simulink model "model_R2019b"  (R2021b)
settings: Solver=FixedStepDiscrete  StartTime=0.0  StopTime=inf  FixedStep=5e-3  RelTol=1e-3
values from neighbouring files (symbols this model uses):
  emin = 0.5    [simulate.m]
  gamma = 0.3    [simulate.m]
  k = 1    [simulate.m]
  omega_max = (pi/180)*300    (= 5.23598775598)    [simulate.m]
  u_max = 1.2    [simulate.m]
libraries: fuzblock x2, simulink x1
settings Model: Creator=mateu  LastModifiedBy=breno-meneses
settings SolverCC: AlgebraicLoopSolver=TrustRegion
settings DebuggingCC: UnconnectedInputMsg=none  UnconnectedOutputMsg=none  UnconnectedLineMsg=none

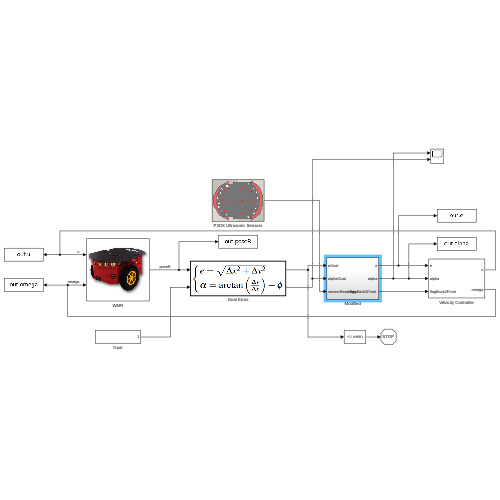
[thumbnail: Simulink's stored preview of the top-level diagram]
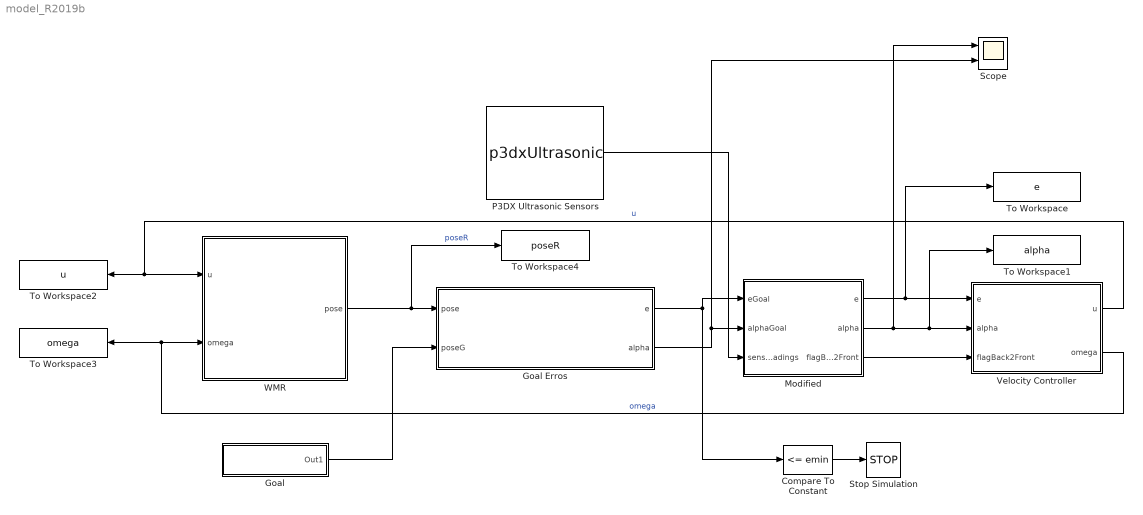
== system model_R2019b ==
  Compare To Constant : simulink/Logic and Bit Operations/Compare To Constant  relop=<=  const=emin  OutDataTypeStr=boolean
  Goal : Subsystem  VariantControl=GOAL_COPPELIA
  Goal Erros : MATLAB Function  TreatAsAtomicUnit=on
  Modified : Subsystem  VariantControl=BC_MODIFIED
  P3DX Ultrasonic Sensors : M-S-Function  FunctionName=p3dxUltrasonic
      mask Display: image('$imagefile'); % Use "Edit Image" on toolstrip to change.
  Scope : Scope  NumInputPorts=2
  Stop Simulation : Stop
  To Workspace : ToWorkspace  VariableName=e  SaveFormat=Timeseries  SampleTime=-1
  To Workspace1 : ToWorkspace  VariableName=alpha  SaveFormat=Timeseries  SampleTime=-1
  To Workspace2 : ToWorkspace  VariableName=u  SaveFormat=Timeseries  SampleTime=-1
  To Workspace3 : ToWorkspace  VariableName=omega  SaveFormat=Timeseries  SampleTime=-1
  To Workspace4 : ToWorkspace  VariableName=poseR  SaveFormat=Timeseries  SampleTime=-1
  Velocity Controller : Subsystem
  WMR : Subsystem  VariantControl=UNICYCLE_COPPELIA
      mask Display: image('$imagefile'); % Use "Edit Image" on toolstrip to change.
  wires:
  WMR/1(pose) -> To Workspace4/1, Goal Erros/1(pose)  "poseR"
  Goal/1(Out1) -> Goal Erros/2(poseG)
  Compare To Constant/1 -> Stop Simulation/1
  Velocity Controller/1(u) -> WMR/1(u), To Workspace2/1  "u"
  Velocity Controller/2(omega) -> WMR/2(omega), To Workspace3/1  "omega"
  Modified/1(e) -> Velocity Controller/1(e), To Workspace/1
  Modified/2(alpha) -> Velocity Controller/2(alpha), To Workspace1/1, Scope/1
  Goal Erros/1(e) -> Modified/1(eGoal), Compare To Constant/1
  Goal Erros/2(alpha) -> Scope/2, Modified/2(alphaGoal)
  P3DX Ultrasonic Sensors/1 -> Modified/3(sensorReadings)
  Modified/3("flagBack2Front ") -> Velocity Controller/3("flagBack2Front ")

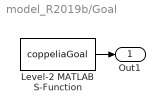
== system model_R2019b/Goal ==
  Level-2 MATLAB S-Function : M-S-Function  FunctionName=coppeliaGoal
  Out1 : Outport
  wires:
  Level-2 MATLAB S-Function/1 -> Out1/1

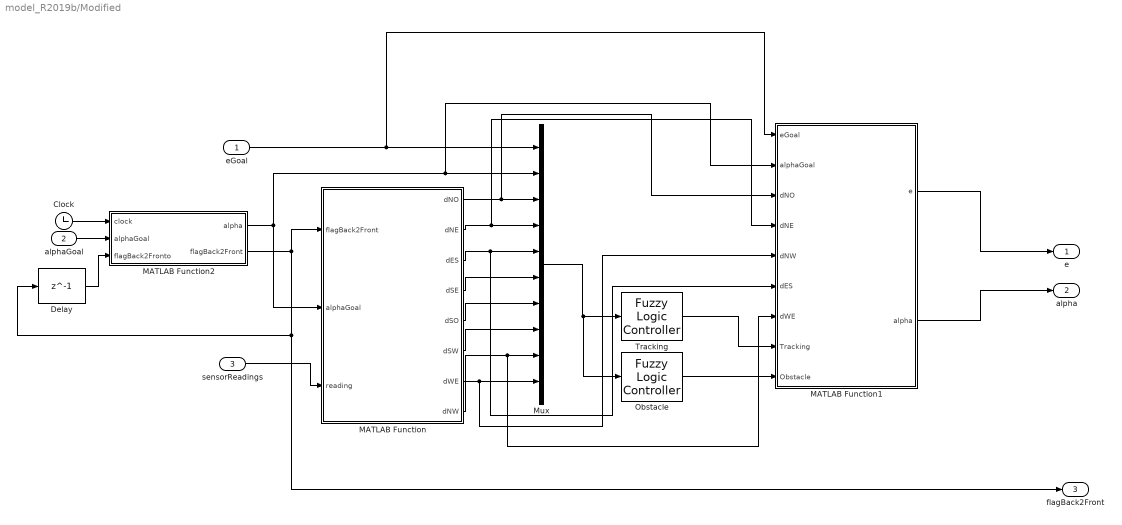
== system model_R2019b/Modified ==
  eGoal : Inport
  alphaGoal : Inport  Port=2
  sensorReadings : Inport  Port=3
  Clock : Clock
  Delay : Delay  DelayLength=1  InputProcessing=Columns as channels (frame based)
  MATLAB Function : MATLAB Function  TreatAsAtomicUnit=on
  MATLAB Function1 : MATLAB Function  TreatAsAtomicUnit=on
  MATLAB Function2 : MATLAB Function  TreatAsAtomicUnit=on
  Mux : Mux  Inputs=10
  "Obstacle " : fuzblock/Fuzzy Logic  Controller  FIS=Obstacle  OutputSampleNumber=101  DataType=double  FuzzifiedInputs=off  RuleFiringStrengths=off  RuleOutputs=off  AggregatedOutputs=off  SimulateUsing=Interpreted execution  OutOfRangeInputValueMessage=warning  NoRuleFiredMessage=warning  EmptyOutputFuzzySetMessage=warning
  Tracking : fuzblock/Fuzzy Logic  Controller  FIS=Tracking  OutputSampleNumber=101  DataType=double  FuzzifiedInputs=off  RuleFiringStrengths=off  RuleOutputs=off  AggregatedOutputs=off  SimulateUsing=Interpreted execution  OutOfRangeInputValueMessage=warning  NoRuleFiredMessage=warning  EmptyOutputFuzzySetMessage=warning
  e : Outport
  alpha : Outport  Port=2
  "flagBack2Front " : Outport  Port=3
  wires:
  sensorReadings/1 -> MATLAB Function/3(reading)
  MATLAB Function/1(dNO) -> MATLAB Function1/3(dNO), Mux/3
  MATLAB Function/2(dNE) -> MATLAB Function1/4(dNE), Mux/4
  MATLAB Function/3(dES) -> MATLAB Function1/6(dES), Mux/5
  MATLAB Function/4(dSE) -> Mux/6
  MATLAB Function/5(dSO) -> Mux/7
  MATLAB Function/6(dSW) -> Mux/8
  MATLAB Function/7(dWE) -> MATLAB Function1/7(dWE), Mux/9
  MATLAB Function/8(dNW) -> MATLAB Function1/5(dNW), Mux/10
  eGoal/1 -> MATLAB Function1/1(eGoal), Mux/1
  MATLAB Function1/2(alpha) -> alpha/1
  MATLAB Function1/1(e) -> e/1
  Tracking/1 -> MATLAB Function1/8(Tracking)
  MATLAB Function2/1(alpha) -> MATLAB Function/2(alphaGoal), MATLAB Function1/2(alphaGoal), Mux/2
  "Obstacle "/1 -> MATLAB Function1/9(Obstacle)
  Mux/1 -> "Obstacle "/1, Tracking/1
  MATLAB Function2/2(flagBack2Front) -> Delay/1, "flagBack2Front "/1, MATLAB Function/1(flagBack2Front)
  alphaGoal/1 -> MATLAB Function2/2(alphaGoal)
  Clock/1 -> MATLAB Function2/1(clock)
  Delay/1 -> MATLAB Function2/3(flagBack2Fronto)

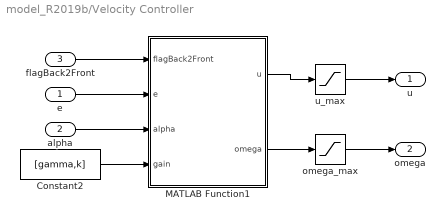
== system model_R2019b/Velocity Controller ==
  e : Inport
  alpha : Inport  Port=2
  "flagBack2Front " : Inport  Port=3
  Constant2 : Constant  Value=[gamma,k]
  MATLAB Function1 : MATLAB Function  TreatAsAtomicUnit=on
  omega_max : Saturate  UpperLimit=omega_max  LowerLimit=-omega_max
  u_max : Saturate  UpperLimit=u_max  LowerLimit=-u_max
  u : Outport
  omega : Outport  Port=2
  wires:
  Constant2/1 -> MATLAB Function1/4(gain)
  omega_max/1 -> omega/1
  u_max/1 -> u/1
  alpha/1 -> MATLAB Function1/3(alpha)
  e/1 -> MATLAB Function1/2(e)
  MATLAB Function1/2(omega) -> omega_max/1
  MATLAB Function1/1(u) -> u_max/1
  "flagBack2Front "/1 -> MATLAB Function1/1(flagBack2Front)

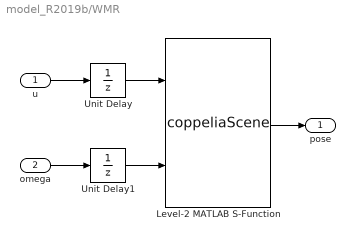
== system model_R2019b/WMR ==
  u : Inport
  omega : Inport  Port=2
  Level-2 MATLAB S-Function : M-S-Function  FunctionName=coppeliaScene
  Unit Delay : UnitDelay  SampleTime=-1  HasFrameUpgradeWarning=on
  Unit Delay1 : UnitDelay  SampleTime=-1  HasFrameUpgradeWarning=on
  pose : Outport
  wires:
  u/1 -> Unit Delay/1
  omega/1 -> Unit Delay1/1
  Level-2 MATLAB S-Function/1 -> pose/1
  Unit Delay/1 -> Level-2 MATLAB S-Function/1
  Unit Delay1/1 -> Level-2 MATLAB S-Function/2

== matlab function model_R2019b/Modified/MATLAB Function ==
  data: flagBack2Front input; alphaGoal input; reading input; dNO output; dNE output; dES output; dSE output; dSO output; dSW output; dWE output; dNW output
function [dNO,dNE,dES,dSE,dSO,dSW,dWE,dNW] = getDistances(flagBack2Front,alphaGoal,reading)

    
if(flagBack2Front)
    dNO = min(reading(12:13));
    dSO = min(reading(4:5));
    dES = min([reading(1),reading(16)]);
    dWE = min(reading(8:9));
    dSE = min(reading(2:3));
    dNW = min(reading(10:11));
    dNE = min(reading(14:15)); 
    dSW = min(reading(6:7));
else
    dNO = min(reading(4:5));
    dSO = min(reading(12:13));
    dES = min(reading(8:9));
    dWE = min([reading(1),reading(16)]);
    dSE = min(reading(10:11));
    dNW = min(reading(2:3));
    dNE = min(reading(6:7));
    dSW = min(reading(14:15));
end

end

== matlab function model_R2019b/Goal Erros ==
  settings: updateMethod=DISCRETE  sampleTime=0.05
  data: pose input; e output; poseG input; alpha output
function [e,alpha] = errors(pose,poseG)

deltaX = poseG(1)-pose(1); deltaY = poseG(2)-pose(2);
phi = pose(3);

e = sqrt(deltaX^2 + deltaY^2);
alpha = atan2(deltaY,deltaX) - phi;

if alpha < -pi
    alpha = alpha + 2*pi;
elseif alpha >= pi
    alpha = alpha - 2*pi;
end

== matlab function model_R2019b/Velocity Controller/MATLAB Function1 ==
  settings: updateMethod=DISCRETE  sampleTime=0.05
  data: flagBack2Front input; e input; u output; alpha input; omega output; gain input
function [u,omega] = control(flagBack2Front,e,alpha,gain)

gamma = gain(1); k = gain(2);

u = gamma*e*cos(alpha);
omega = k*alpha + gamma*cos(alpha)*sin(alpha);

if(flagBack2Front)
    u = -u;
end

== matlab function model_R2019b/Modified/MATLAB Function1 ==
  data: eGoal input; alphaGoal input; dNO input; dNE input; dNW input; dES input; dWE input; e output; Tracking input; Obstacle input; alpha output
function [e, alpha]  = alterStates(eGoal,alphaGoal,dNO,dNE,dNW,dES,dWE,Tracking, Obstacle)
 
    if (dNO<1.5 || dNE<1.5 || dNW<1.5)
        e=Obstacle(1);
        alpha=Obstacle(2);
    elseif dNO>=2 && (dES<1.5 || dWE<1.5)  
        e=Tracking(1);
        alpha=Tracking(2);
    else   
        e=eGoal;
        alpha=alphaGoal;
    end
  
end

== matlab function model_R2019b/Modified/MATLAB Function2 ==
  data: clock input; alphaGoal input; alpha output; flagBack2Front output; flagBack2Fronto input
function [alpha, flagBack2Front] = flagBack2Front(clock, alphaGoal, flagBack2Fronto)
function [alpha, flagBack2Front] = flagBack2Front(clock, alphaGoal, flagBack2Fronto)
function [alpha, flagBack2Front] = flagBack2Front(clock, alphaGoal, flagBack2Fronto)
function [alpha, flagBack2Front] = flagBack2Front(clock, alphaGoal, flagBack2Fronto)
function [alpha,flagBack2Front] = flagBack2Front(clock,alphaGoal,flagBack2Fronto)

if(clock == 0)
    alphaGoalnorm = abs(rad2deg(alphaGoal));
    flagBack2Front = double(alphaGoalnorm > 90);
else
    flagBack2Front = flagBack2Fronto;
end

if(alphaGoal > 0 && flagBack2Front)
    alpha=alphaGoal-pi;
elseif (alphaGoal < 0 && flagBack2Front)
    alpha=alphaGoal+pi;
else
    alpha=alphaGoal;
end
